simulink model "sldemo_engine"  (R2025a)
settings: Solver=ode45  StartTime=0.0  StopTime=3  RelTol=1e-3  AbsTol=1e-6
Description:
  | Modeling Engine Timing Using Triggered Subsystems
  | 
  | This example shows how to model of a four-cylinder spark ignition engine
  | and shows Simulink(R) capabilities to model an internal combustion
  | engine from the throttle to the crankshaft output. We used well-defined
  | physical principles supplemented, where appropriate, with empirical
  | relationships that describe the systems dynamic behavior without
  | introducing unnecessary complexity.
settings Model: ExtModeTrigMode=oneshot  ExtModeArmWhenConnect=off  ExtModeAutoUpdateStatusClock=off  Creator=The MathWorks, Inc.
settings SolverCC: AutoScaleAbsTol=off  AlgebraicLoopSolver=TrustRegion
settings DataIOCC: ExternalInput=[]  InitialState=[]  SaveFormat=Array  SignalLogging=off  SaveTime=off  StateSaveName=x  TimeSaveName=t  SignalLoggingName=sldemo_engine_output
settings OptimizationCC: BlockReduction=off  ExpressionDepthLimit=2147483647.0  InitFltsAndDblsToZero=on  LifeSpan=inf  BufferReusableBoundary=off
settings DebuggingCC: SaveWithParameterizedLinksMsg=none  SignalResolutionControl=TryResolveAllWithWarning  MultiTaskDSMMsg=warning  MultiTaskCondExecSysMsg=none  SigSpecEnsureSampleTimeMsg=none  IntegerOverflowMsg=none  FcnCallInpInsideContextMsg=warning  UnconnectedInputMsg=warning  UnconnectedOutputMsg=warning  UnconnectedLineMsg=warning  BusObjectLabelMismatch=none  StateNameClashWarn=warning  SFUnexpectedBacktrackingDiag=warning  SFNoUnconditionalDefaultTransitionDiag=warning  SFExecutionAtInitializationDiag=none  IntegerSaturationMsg=none  ArithmeticOperatorsInVariantConditions=warning
settings HardwareCC: ProdBitPerPointer=32.0  ProdBitPerSizeT=32.0  ProdBitPerPtrDiffT=32.0  ProdLargestAtomicFloat=None  ProdIntDivRoundTo=Undefined  ProdEndianess=Unspecified  ProdWordSize=32.0  ProdHWDeviceType=32-bit Generic
settings ModelReferenceCC: EnableRefExpFcnMdlSchedulingChecks=on  PropagateSignalLabelsOutOfModel=off
settings SFSimCC: SimUseLocalCustomCode=off  CustomCodeUndefinedFunction=UseInterfaceOnly
settings RTWCC: RTWUseLocalCustomCode=off  GPUComputeCapability=3.5
settings CodeAppCC: StateflowObjectComments=on
settings GRTTargetCC: TargetFcnLib=ansi_tfl_tmw.mat  TargetLangStandard=C89/C90 (ANSI)  CombineOutputUpdateFcns=off  GRTInterface=on
settings ConfigComp: CovMetricSettings=d  CovSaveCumulativeToWorkspaceVar=on  CovSaveSingleToWorkspaceVar=on  CovExternalEMLEnable=off

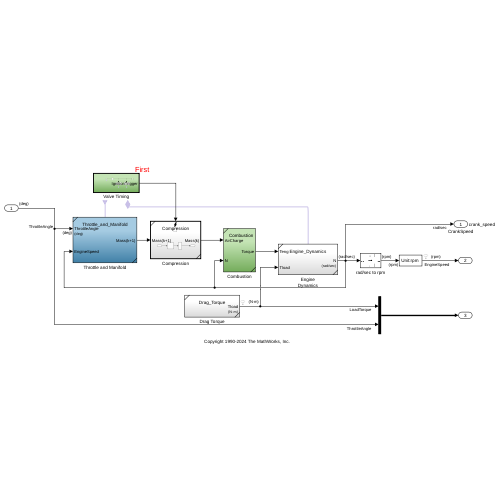
[thumbnail: Simulink's stored preview of the top-level diagram]
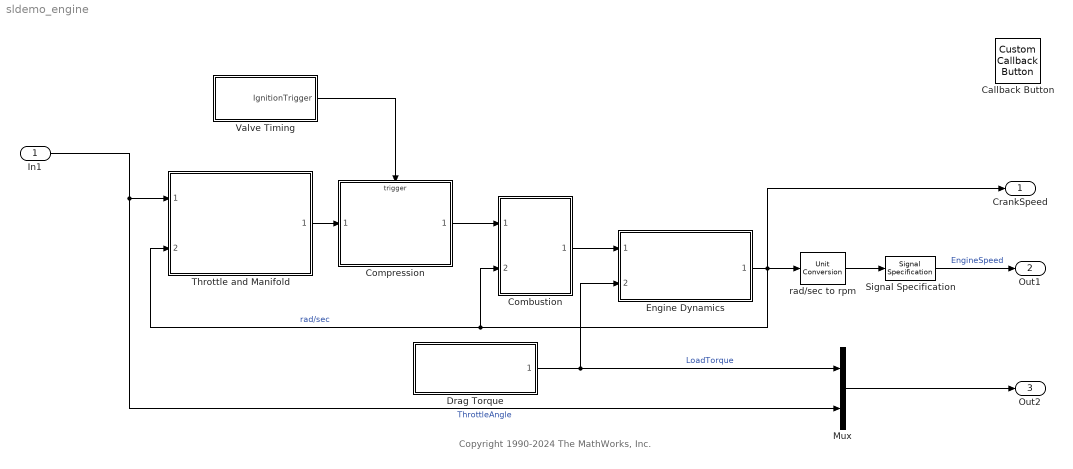
== system sldemo_engine ==
  note: Copyright 1990-2024 The MathWorks, Inc.
  In1 : Inport
  Callback Button : CustomCallbackButton  Configuration="{\"components\":[{\"name\":\"BackgroundImageComponent\",\"settings\":{\"image\":{\"size\":[0,0],\"src\":\"default\",\"srcOrientation\":\"Right\"},\"position\":[0,0,1,1]}},{\"name\":\"ButtonStateComponent\",\"settings\":{\"buttonType\":\"momentary\",\"clickFcn\":\"showExample(\\\"simulink_automotive\\/ModelingEngineTimingUsingTriggeredSubsystemsExample\\\")\",\"onValue\":1,\"position\":[0,0,1,1],\"pressDelay\":\"500\",\"pressFcn\":\"\",\"repeatInterval\":\"0\",\"states\":[{\"horizontalAlignment\":\"center\",\"image\":{\"position\":[0,0,1,1],\"size\":[1,1],\"src\":\"default\",\"srcOrientation\":\"Right\"},\"label\":{\"color\":[0.01176470588,0.01176470588,0.01176470588,1],\"icon\":{\"size\":[0,0],\"src\":\"default\",\"srcOrientation\":\"Right\"},\"iconPlacement\":\"left\",\"opacity\":1,\"show\":true,\"text\":{\"content\":\"?\",\"font\":\"Helvetica\"}},\"labelOffset\":[0,0],\"verticalAlignment\":\"middle\"},{\"horizontalAlignment\":\"center\",\"image\":{\"position\":[0,0,1,1],\"size\":[1,1],\"src\":\"default\",\"srcOrientation\":\"Right\"},\"label\":{\"color\":[0.01176470588,0.01176470588,0.01176470588,1],\"icon\":{\"size\":[0,0],\"src\":\"default\",\"srcOrientation\":\"Right\"},\"iconPlacement\":\"left\",\"opacity\":1,\"show\":true,\"text\":{\"content\":\"?\",\"font\":\"Helvetica\"}},\"labelOffset\":[0,0],\"verticalAlignment\":\"middle\"},{\"horizontalAlignment\":\"center\",\"image\":{\"position\":[0,0,1,1],\"size\":[1,1],\"src\":\"default\",\"srcOrientation\":\"Right\"},\"label\":{\"color\":[0.01176470588,0.01176470588,0.01176470588,1],\"icon\":{\"size\":[0,0],\"src\":\"default\",\"srcOrientation\":\"Right\"},\"iconPlacement\":\"left\",\"opacity\":1,\"show\":true,\"text\":{\"content\":\"?\",\"font\":\"Helvetica\"}},\"labelOffset\":[0,0],\"verticalAlignment\":\"middle\"},{\"horizontalAlignment\":\"center\",\"image\":{\"position\":[0,0,1,1],\"size\":[1,1],\"src\":\"default\",\"srcOrientation\":\"Right\"},\"label\":{\"color\":[0.01176470588,0.01176470588,0.01176470588,1],\"icon\":{\"size\":[0,0],\"src\":\"default\",\"srcOrientation\":\"Right\"},\"iconPlacement\":\"left\",\"opacity\":1,\"show\":true,\"text\":{\"content\":\"?\",\"font\":\"Helvetica\"}},\"labelOffset\":[0,0],\"verticalAlignment\":\"middle\"}]}},{\"name\":\"ForegroundImageComponent\",\"settings\":{\"image\":{\"size\":[0,0],\"src\":\"default\",\"srcOrientation\":\"Right\"},\"isForeground\":1,\"position\":[0,0,1,1]}}],\"derived\":{\"blockParameters\":{\"AutoActivate\":true,\"ButtonText\":\"?\",\"ButtonType\":\"Momentary\",\"ClickFcn\":\"showExample(\\\"simulink_automotive\\/ModelingEngineTimingUsingTriggeredSubsystemsExample\\\")\",\"OnValue\":1,\"PressDelay\":\"500\",\"PressFcn\":\"\",\"RepeatInterval\":\"0\",\"fixedAspectRatio\":\"off\"}},\"settings\":{\"BindingType\":\"standalone\",\"autoActivate\":true,\"backgroundColor\":[244,244,244,1],\"backgroundOffset\":0.2,\"backgroundOpacity\":1,\"fixedAspectRatio\":\"off\",\"foregroundColor\":[0.01176470588,0.01176470588,0.01176470588,1],\"migratedFromLegacy\":true,\"useBackgroundColor\":true,\"variant\":\"callback\",\"version\":\"R2025a\"},\"type\":\"Button\"}"  CustomBackgroundColor="{\"color\":[0.9568627451,0.9568627451,0.9568627451],\"show\":true}"
  Combustion : Subsystem  ReferencedSubsystem=Combustion
  Compression : Subsystem  TreatAsAtomicUnit=on  ReferencedSubsystem=Compression
  Drag Torque : Subsystem  ReferencedSubsystem=Drag_Torque
  Engine Dynamics : Subsystem  ReferencedSubsystem=Engine_Dynamics
  Mux : Mux  Inputs=2
  Signal Specification : SignalSpecification  Unit=rpm
  Throttle and Manifold : Subsystem  ReferencedSubsystem=Throttle_and_Manifold
  Valve Timing : Subsystem  ExecutionOrder=First  TreatAsAtomicUnit=on
  rad/sec to rpm : UnitConversion
  CrankSpeed : Outport  SignalName=crank_speed  InitialOutput=0  VectorParamsAs1DForOutWhenUnconnected=off
  Out1 : Outport  Port=2
  Out2 : Outport  Port=3
  wires:
  Valve Timing/1(IgnitionTrigger) -> Compression/Trigger
  Throttle and Manifold/1 -> Compression/1
  Engine Dynamics/1 -> Combustion/2, Throttle and Manifold/2, CrankSpeed/1, rad/sec to rpm/1  "rad/sec"
  Mux/1 -> Out2/1
  Combustion/1 -> Engine Dynamics/1
  Compression/1 -> Combustion/1
  In1/1 -> Throttle and Manifold/1, Mux/2  "ThrottleAngle"
  rad/sec to rpm/1 -> Signal Specification/1
  Drag Torque/1 -> Engine Dynamics/2, Mux/1  "LoadTorque"
  Signal Specification/1 -> Out1/1  "EngineSpeed"

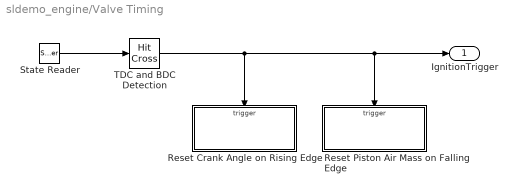
== system sldemo_engine/Valve Timing ==
  Reset Crank Angle on Rising Edge : Subsystem  TreatAsAtomicUnit=on
  Reset Piston Air Mass on Falling Edge : Subsystem  TreatAsAtomicUnit=on
  State Reader : StateReader  StateOwnerBlock=../../Engine Dynamics/Crank Integrator  StateName=CrankAngle
  TDC and BDC Detection : HitCross  HitCrossingOffset=pi  HitCrossingDirection=rising
  IgnitionTrigger : Outport
  wires:
  State Reader/1 -> TDC and BDC Detection/1
  TDC and BDC Detection/1 -> IgnitionTrigger/1, Reset Piston Air Mass on Falling Edge/Trigger, Reset Crank Angle on Rising Edge/Trigger

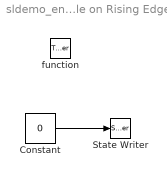
== system sldemo_engine/Valve Timing/Reset Crank Angle on Rising Edge ==
  function : TriggerPort  VariantControl=(inherit)  InitialTriggerSignalState=zero
  Constant : Constant  Value=0
  State Writer : StateWriter  StateOwnerBlock=../../../Engine Dynamics/Crank Integrator  StateName=CrankAngle
  wires:
  Constant/1 -> State Writer/1

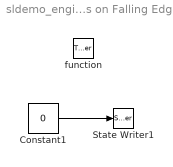
== system sldemo_engine/Valve Timing/Reset Piston Air Mass on Falling Edge ==
  function : TriggerPort  TriggerType=falling  VariantControl=(inherit)  InitialTriggerSignalState=zero
  Constant1 : Constant  Value=0
  State Writer1 : StateWriter  StateOwnerBlock=../../../Throttle and Manifold/PistonAirMass
  wires:
  Constant1/1 -> State Writer1/1
